simulink model "kinovaMicoSimscapeModel"  (R2021b)
settings: Solver=VariableStepAuto  StartTime=0.0  StopTime=0.3  FixedStep=0.01  RelTol=1e-3
PostLoadFcn:
  | micoRigidBodyTreeCreation;
  | IC=deg2rad([-90,180,180,0,0,0]);
  | interactiveHomePosition=deg2rad([-90 90 177.5 90 0 0]');
  | load("./KinovaMicoSimscapeVariantConfigurations.mat");
values from neighbouring files (symbols this model uses):
  micoCandlePosition = deg2rad([0,180,180,0,0,0])    [KinovaMicoSimscapeInitializeScript.m]    (also in generatingRandomTrajectory.m)
  ViaPointsTaskSpace = [ViaPointsTaskSpace;[[pi;0;pi],[pi;0;pi],[pi;0;pi],[pi;0;pi],[0;0;0],[0;0;0],[pi;0;pi]]]    [KinovaMicoSimscapeInitializeScript.m]    (also in generatingRandomTrajectory.m = [ViaPointsTaskSpace;zeros(3,7)])
undefined symbols (not defined in the file or in its folder): Mico, ViaPointsJointSpace, X, Y, Z
libraries: sm_lib x26, nesl_utility x19, robotcorelib x4, robotmaniplib x3, pid_lib x2
(part 2 of 50)

== system kinovaMicoSimscapeModel/StateErrorNorm/TaskSpaceError/Compute dqError ==
  dqd : Inport
  dq : Inport  Port=2
  Dot Product : DotProduct  InputSameDT=on  OutDataTypeStr=Inherit: Inherit via internal rule
  Sqrt : Sqrt  SaturateOnIntegerOverflow=on
  Subsystem : Subsystem  Commented=on
  Sum : Sum  Inputs=|+-
  dq_error : Outport
  wires:
  Sqrt/1 -> dq_error/1
  dq/1 -> Sum/2
  dqd/1 -> Sum/1
  Dot Product/1 -> Sqrt/1
  Sum/1 -> Dot Product/1, Dot Product/2

== system kinovaMicoSimscapeModel/StateErrorNorm/TaskSpaceError/Compute qError ==
  qd : Inport
  q : Inport  Port=2
  Dot Product : DotProduct  InputSameDT=on  OutDataTypeStr=Inherit: Inherit via internal rule
  Sqrt : Sqrt  SaturateOnIntegerOverflow=on
  Sum : Sum  Inputs=|+-
  q_error : Outport
  wires:
  Sum/1 -> Dot Product/2, Dot Product/1
  Dot Product/1 -> Sqrt/1
  qd/1 -> Sum/1
  q/1 -> Sum/2
  Sqrt/1 -> q_error/1

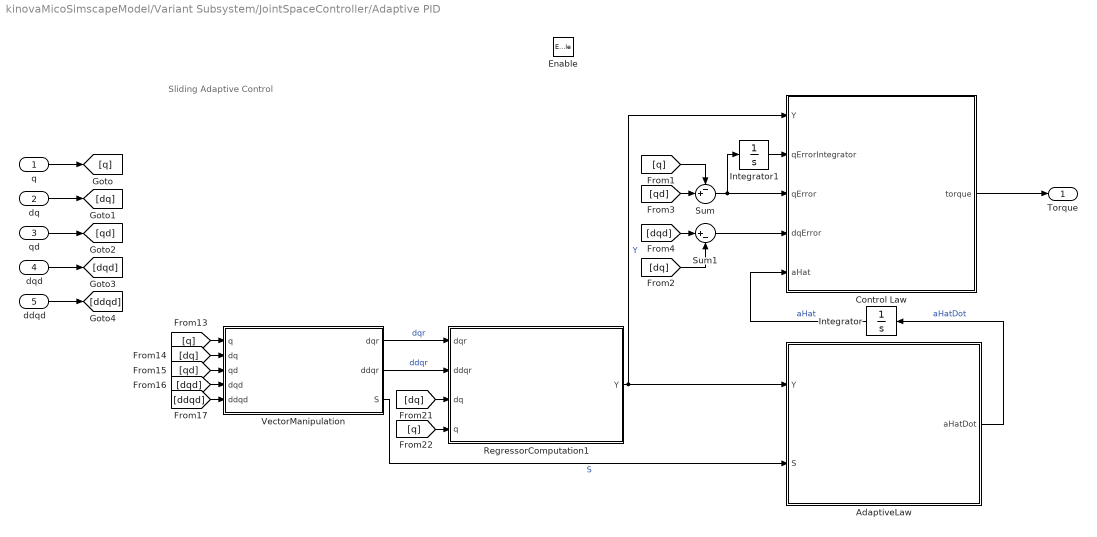
== system kinovaMicoSimscapeModel/Variant Subsystem/JointSpaceController/Adaptive PID ==
  note: Sliding Adaptive Control
  q : Inport
  dq : Inport  Port=2
  qd : Inport  Port=3
  dqd : Inport  Port=4
  ddqd : Inport  Port=5
  Enable : EnablePort
  AdaptiveLaw : MATLAB Function  TreatAsAtomicUnit=on
  Control Law : MATLAB Function  TreatAsAtomicUnit=on
  Integrator : Integrator
  Integrator1 : Integrator
  RegressorComputation1 : MATLAB Function  TreatAsAtomicUnit=on
  Sum : Sum  Inputs=-+|
  Sum1 : Sum  Inputs=|+-
  VectorManipulation : MATLAB Function  TreatAsAtomicUnit=on
  Torque : Outport
  wires:
  VectorManipulation/2(ddqr) -> RegressorComputation1/2(ddqr)  "ddqr"
  [qd] -> VectorManipulation/3(qd)
  VectorManipulation/3(S) -> AdaptiveLaw/2(S)  "S"
  [dqd] -> VectorManipulation/4(dqd)
  [ddqd] -> VectorManipulation/5(ddqd)
  [dq] -> RegressorComputation1/3(dq)
  [q] -> VectorManipulation/1(q)
  RegressorComputation1/1(Y) -> AdaptiveLaw/1(Y), Control Law/1(Y)  "Y"
  [dq] -> VectorManipulation/2(dq)
  Integrator/1 -> Control Law/5(aHat)  "aHat"
  [q] -> RegressorComputation1/4(q)
  VectorManipulation/1(dqr) -> RegressorComputation1/1(dqr)  "dqr"
  AdaptiveLaw/1(aHatDot) -> Integrator/1  "aHatDot"
  Control Law/1(torque) -> Torque/1
  q/1 -> [q]
  dq/1 -> [dq]
  qd/1 -> [qd]
  dqd/1 -> [dqd]
  ddqd/1 -> [ddqd]
  Sum/1 -> Integrator1/1, Control Law/3(qError)
  Integrator1/1 -> Control Law/2(qErrorIntegrator)
  [qd] -> Sum/2
  [q] -> Sum/1
  [dqd] -> Sum1/1
  [dq] -> Sum1/2
  Sum1/1 -> Control Law/4(dqError)

== system kinovaMicoSimscapeModel/Variant Subsystem/JointSpaceController/Enabled Subsystem ==
  q : Inport
  G_RNE : MATLAB Function  TreatAsAtomicUnit=on
  G : Outport
  wires:
  q/1 -> G_RNE/1(q)
  G_RNE/1(G) -> G/1  "gravity"

== system kinovaMicoSimscapeModel/Variant Subsystem/JointSpaceController/HybridImpedanceVelocityControl ==
  q : Inport
  dq : Inport  Port=2
  ddq : Inport  Port=3
  qd : Inport  Port=4
  dqd : Inport  Port=5
  ddqd : Inport  Port=6
  f : Inport  Port=7
  G : Inport  Port=8
  Enable : EnablePort
  C_RNE_SKEWSYMETRIC : MATLAB Function  TreatAsAtomicUnit=on
  Display : Display
  H_RNE : MATLAB Function  TreatAsAtomicUnit=on
  Hybrid Impedance Velocity Control : MATLAB Function  TreatAsAtomicUnit=on
  torque : Outport
  wires:
  ddq/1 -> Hybrid Impedance Velocity Control/3(ddq)
  Hybrid Impedance Velocity Control/1(torque) -> torque/1
  q/1 -> [q], Hybrid Impedance Velocity Control/1(q)
  dq/1 -> [dq], Hybrid Impedance Velocity Control/2(dq)
  qd/1 -> Hybrid Impedance Velocity Control/4(qd)
  dqd/1 -> Hybrid Impedance Velocity Control/5(dqd)
  ddqd/1 -> Hybrid Impedance Velocity Control/6(ddqd)
  f/1 -> Hybrid Impedance Velocity Control/7(f)
  H_RNE/1(M) -> Hybrid Impedance Velocity Control/8(H)  "mass"
  [q] -> H_RNE/1(q), C_RNE_SKEWSYMETRIC/1(q)
  [dq] -> C_RNE_SKEWSYMETRIC/2(dq)
  C_RNE_SKEWSYMETRIC/1(C) -> Hybrid Impedance Velocity Control/9(C)
  G/1 -> Hybrid Impedance Velocity Control/10(G)
  Hybrid Impedance Velocity Control/2(test) -> Display/1

== system kinovaMicoSimscapeModel/Variant Subsystem/JointSpaceController/Inverse Dynamics ==
  note: Inverse Dynamics
  q : Inport
  dq : Inport  Port=2
  qd : Inport  Port=3
  dqd : Inport  Port=4
  ddqd : Inport  Port=5
  G : Inport  Port=6
  Enable : EnablePort
  C_RNE_SKEWSYMETRIC : MATLAB Function  TreatAsAtomicUnit=on
  H_RNE : MATLAB Function  TreatAsAtomicUnit=on
  Inverse Dynamics : MATLAB Function  TreatAsAtomicUnit=on
  Matrix Multiply : Product  Multiplication=Matrix(*)
  Torque : Outport
  wires:
  ddqd/1 -> [ddqd]
  dqd/1 -> [dqd]
  qd/1 -> [qd]
  dq/1 -> [dq]
  q/1 -> [q]
  Inverse Dynamics/1(torque) -> Torque/1  "ComputedTorque"
  [q] -> H_RNE/1(q), C_RNE_SKEWSYMETRIC/1(q)
  [dq] -> C_RNE_SKEWSYMETRIC/2(dq)
  C_RNE_SKEWSYMETRIC/1(C) -> Matrix Multiply/1
  [dq] -> Matrix Multiply/2
  [q] -> Inverse Dynamics/4(q)
  [dq] -> Inverse Dynamics/5(dq)
  [qd] -> Inverse Dynamics/6(qd)
  [dqd] -> Inverse Dynamics/7(dqd)
  [ddqd] -> Inverse Dynamics/8(ddqd)
  H_RNE/1(M) -> Inverse Dynamics/1(M)  "mass"
  Matrix Multiply/1 -> Inverse Dynamics/2(Cdq)  "customCdq"
  G/1 -> Inverse Dynamics/3(G)

== system kinovaMicoSimscapeModel/Variant Subsystem/JointSpaceController/PD + Gravity ==
  note: Inputs
  note: PD + Gravity Controller
  q : Inport
  dq : Inport  Port=2
  qd : Inport  Port=3
  dqd : Inport  Port=4
  ddqd : Inport  Port=5
  G : Inport  Port=6
  Enable : EnablePort
  Gain : Gain  Gain=diag([25 25 25 15 15 15])  Multiplication=Matrix(K*u)
  Gain2 : Gain  Gain=diag([5 5 5 2 2 2])  Multiplication=Matrix(K*u)
  Sum : Sum  Inputs=|+-
  Sum1 : Sum  Inputs=|++
  Sum3 : Sum  Inputs=|+-
  Terminator : Terminator
  Terminator2 : Terminator
  Torque : Outport
  wires:
  Sum1/1 -> Torque/1
  dqd/1 -> Terminator2/1
  ddqd/1 -> Terminator/1
  qd/1 -> [qd]
  dq/1 -> [dq]
  q/1 -> [q]
  [q] -> Sum/2
  [dq] -> Gain2/1
  [qd] -> Sum/1
  Sum/1 -> Gain/1
  Gain/1 -> Sum3/1
  Gain2/1 -> Sum3/2
  Sum3/1 -> Sum1/1
  G/1 -> Sum1/2  "gravity"

== system kinovaMicoSimscapeModel/Variant Subsystem/JointSpaceController/PID ==
  note: Damping + Gravity Controller
  q : Inport
  dq : Inport  Port=2
  qd : Inport  Port=3
  dqd : Inport  Port=4
  ddqd : Inport  Port=5
  G : Inport  Port=6
  Enable : EnablePort
  Gain2 : Gain  Gain=0.1*ones(6,1)
  Gain3 : Gain  Gain=0.65*diag([25 25 25 8 8 8])  Multiplication=Matrix(K*u)
  Gain4 : Gain  Gain=0.25*diag([5 4 3 2 1.5 1.5])  Multiplication=Matrix(K*u)
  Integrator : Integrator
  Sum : Sum  Inputs=|+-
  Sum1 : Sum  Inputs=++++
  Sum2 : Sum  Inputs=|+-
  Terminator : Terminator
  Torque : Outport
  wires:
  Sum1/1 -> Torque/1
  dqd/1 -> [dqd]
  ddqd/1 -> Terminator/1
  qd/1 -> [qd]
  dq/1 -> [dq]
  q/1 -> [q]
  [qd] -> Sum/1
  [q] -> Sum/2
  [dqd] -> Sum2/1
  [dq] -> Sum2/2
  Sum/1 -> Gain3/1, Integrator/1
  Gain3/1 -> Sum1/2
  Sum2/1 -> Gain4/1
  Gain4/1 -> Sum1/3
  Integrator/1 -> Gain2/1
  Gain2/1 -> Sum1/1
  G/1 -> Sum1/4  "gravity"

== system kinovaMicoSimscapeModel/Variant Subsystem/JointSpaceController/Sliding Adaptive Control ==
  note: Sliding Adaptive Control
  q : Inport
  dq : Inport  Port=2
  qd : Inport  Port=3
  dqd : Inport  Port=4
  ddqd : Inport  Port=5
  Enable : EnablePort
  AdaptiveLaw : MATLAB Function  TreatAsAtomicUnit=on
  Control Law : MATLAB Function  TreatAsAtomicUnit=on
  Integrator : Integrator
  RegressorComputation : MATLAB Function  Commented=on  TreatAsAtomicUnit=on
  RegressorComputation1 : MATLAB Function  TreatAsAtomicUnit=on
  VectorManipulation : MATLAB Function  TreatAsAtomicUnit=on
  torqueDelayStuff : Subsystem  Commented=on
  Torque : Outport
  wires:
  ddqd/1 -> [ddqd]
  dqd/1 -> [dqd]
  qd/1 -> [qd]
  dq/1 -> [dq]
  q/1 -> [q]
  Control Law/1(torque) -> Torque/1  "AdaptiveTorque"
  AdaptiveLaw/1(aHatDot) -> Integrator/1  "aHatDot"
  VectorManipulation/2(dqr) -> RegressorComputation1/1(dqr)  "dqr"
  [q] -> RegressorComputation1/4(q)
  Integrator/1 -> Control Law/3(aHat)  "aHat"
  [dq] -> VectorManipulation/2(dq)
  RegressorComputation1/1(Y) -> Control Law/2(Y), AdaptiveLaw/1(Y)  "Y"
  [q] -> VectorManipulation/1(q)
  [dq] -> RegressorComputation1/3(dq)
  [ddqd] -> VectorManipulation/5(ddqd)
  [dqd] -> VectorManipulation/4(dqd)
  VectorManipulation/1(S) -> AdaptiveLaw/2(S), Control Law/1(S)  "S"
  [qd] -> VectorManipulation/3(qd)
  VectorManipulation/3(ddqr) -> RegressorComputation1/2(ddqr)  "ddqr"

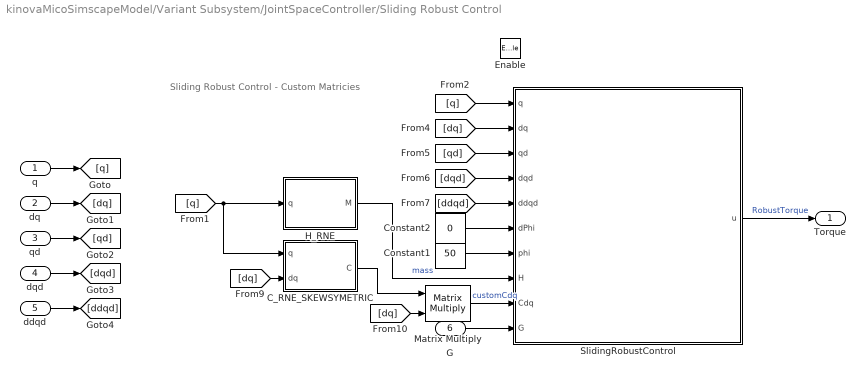
== system kinovaMicoSimscapeModel/Variant Subsystem/JointSpaceController/Sliding Robust Control ==
  note: Sliding Robust Control - Custom Matricies
  q : Inport
  dq : Inport  Port=2
  qd : Inport  Port=3
  dqd : Inport  Port=4
  ddqd : Inport  Port=5
  G : Inport  Port=6
  Enable : EnablePort
  C_RNE_SKEWSYMETRIC : MATLAB Function  TreatAsAtomicUnit=on
  Constant1 : Constant  Value=50
  Constant2 : Constant  Value=0
  H_RNE : MATLAB Function  TreatAsAtomicUnit=on
  Matrix Multiply : Product  Multiplication=Matrix(*)
  SlidingRobustControl : MATLAB Function  TreatAsAtomicUnit=on
  Torque : Outport
  wires:
  [dqd] -> SlidingRobustControl/4(dqd)
  [dq] -> Matrix Multiply/2
  C_RNE_SKEWSYMETRIC/1(C) -> Matrix Multiply/1
  Matrix Multiply/1 -> SlidingRobustControl/9(Cdq)  "customCdq"
  [qd] -> SlidingRobustControl/3(qd)
  [dq] -> C_RNE_SKEWSYMETRIC/2(dq)
  [ddqd] -> SlidingRobustControl/5(ddqd)
  Constant2/1 -> SlidingRobustControl/6(dPhi)
  [q] -> SlidingRobustControl/1(q)
  H_RNE/1(M) -> SlidingRobustControl/8(H)  "mass"
  Constant1/1 -> SlidingRobustControl/7(phi)
  [dq] -> SlidingRobustControl/2(dq)
  [q] -> H_RNE/1(q), C_RNE_SKEWSYMETRIC/1(q)
  SlidingRobustControl/1(u) -> Torque/1  "RobustTorque"
  q/1 -> [q]
  dq/1 -> [dq]
  qd/1 -> [qd]
  dqd/1 -> [dqd]
  ddqd/1 -> [ddqd]
  G/1 -> SlidingRobustControl/10(G)

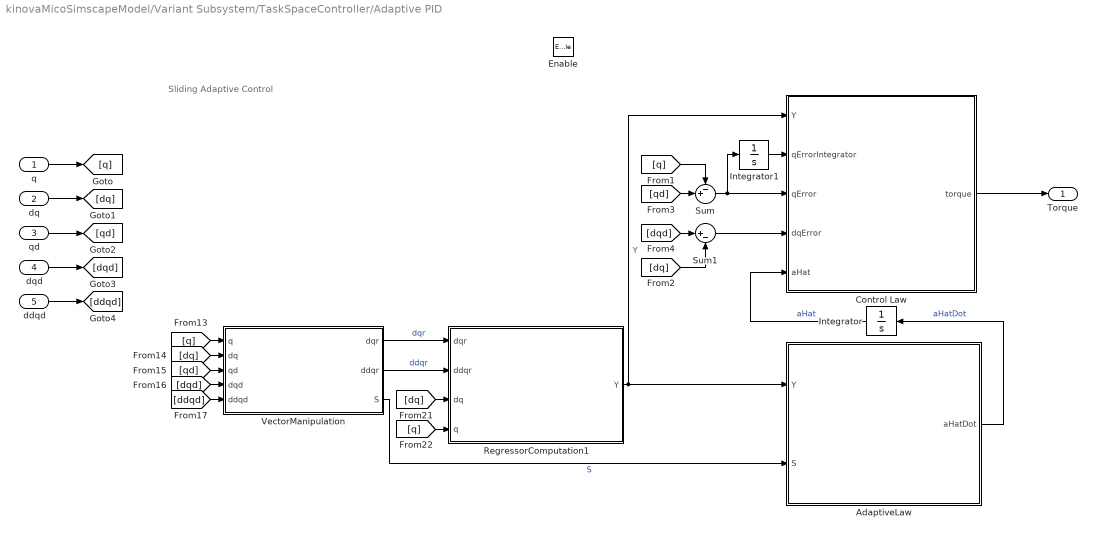
== system kinovaMicoSimscapeModel/Variant Subsystem/TaskSpaceController/Adaptive PID ==
  note: Sliding Adaptive Control
  q : Inport
  dq : Inport  Port=2
  qd : Inport  Port=3
  dqd : Inport  Port=4
  ddqd : Inport  Port=5
  Enable : EnablePort
  AdaptiveLaw : MATLAB Function  TreatAsAtomicUnit=on
  Control Law : MATLAB Function  TreatAsAtomicUnit=on
  Integrator : Integrator
  Integrator1 : Integrator
  RegressorComputation1 : MATLAB Function  TreatAsAtomicUnit=on
  Sum : Sum  Inputs=-+|
  Sum1 : Sum  Inputs=|+-
  VectorManipulation : MATLAB Function  TreatAsAtomicUnit=on
  Torque : Outport
  wires:
  Sum1/1 -> Control Law/4(dqError)
  [dq] -> Sum1/2
  [dqd] -> Sum1/1
  [q] -> Sum/1
  [qd] -> Sum/2
  Integrator1/1 -> Control Law/2(qErrorIntegrator)
  Sum/1 -> Control Law/3(qError), Integrator1/1
  ddqd/1 -> [ddqd]
  dqd/1 -> [dqd]
  qd/1 -> [qd]
  dq/1 -> [dq]
  q/1 -> [q]
  Control Law/1(torque) -> Torque/1
  AdaptiveLaw/1(aHatDot) -> Integrator/1  "aHatDot"
  VectorManipulation/1(dqr) -> RegressorComputation1/1(dqr)  "dqr"
  [q] -> RegressorComputation1/4(q)
  Integrator/1 -> Control Law/5(aHat)  "aHat"
  [dq] -> VectorManipulation/2(dq)
  RegressorComputation1/1(Y) -> Control Law/1(Y), AdaptiveLaw/1(Y)  "Y"
  [q] -> VectorManipulation/1(q)
  [dq] -> RegressorComputation1/3(dq)
  [ddqd] -> VectorManipulation/5(ddqd)
  [dqd] -> VectorManipulation/4(dqd)
  VectorManipulation/3(S) -> AdaptiveLaw/2(S)  "S"
  [qd] -> VectorManipulation/3(qd)
  VectorManipulation/2(ddqr) -> RegressorComputation1/2(ddqr)  "ddqr"

== system kinovaMicoSimscapeModel/Variant Subsystem/TaskSpaceController/Enabled Subsystem ==
  q : Inport
  G_RNE : MATLAB Function  TreatAsAtomicUnit=on
  G : Outport
  wires:
  G_RNE/1(G) -> G/1  "gravity"
  q/1 -> G_RNE/1(q)

== system kinovaMicoSimscapeModel/Variant Subsystem/TaskSpaceController/HybridImpedanceVelocityControl ==
  q : Inport
  dq : Inport  Port=2
  ddq : Inport  Port=3
  qd : Inport  Port=4
  dqd : Inport  Port=5
  ddqd : Inport  Port=6
  f : Inport  Port=7
  G : Inport  Port=8
  Enable : EnablePort
  C_RNE_SKEWSYMETRIC : MATLAB Function  TreatAsAtomicUnit=on
  Display : Display
  H_RNE : MATLAB Function  TreatAsAtomicUnit=on
  Hybrid Impedance Velocity Control : MATLAB Function  TreatAsAtomicUnit=on
  torque : Outport
  wires:
  Hybrid Impedance Velocity Control/2(test) -> Display/1
  G/1 -> Hybrid Impedance Velocity Control/10(G)
  C_RNE_SKEWSYMETRIC/1(C) -> Hybrid Impedance Velocity Control/9(C)
  [dq] -> C_RNE_SKEWSYMETRIC/2(dq)
  [q] -> C_RNE_SKEWSYMETRIC/1(q), H_RNE/1(q)
  H_RNE/1(M) -> Hybrid Impedance Velocity Control/8(H)  "mass"
  f/1 -> Hybrid Impedance Velocity Control/7(f)
  ddqd/1 -> Hybrid Impedance Velocity Control/6(ddqd)
  dqd/1 -> Hybrid Impedance Velocity Control/5(dqd)
  qd/1 -> Hybrid Impedance Velocity Control/4(qd)
  dq/1 -> Hybrid Impedance Velocity Control/2(dq), [dq]
  q/1 -> Hybrid Impedance Velocity Control/1(q), [q]
  Hybrid Impedance Velocity Control/1(torque) -> torque/1
  ddq/1 -> Hybrid Impedance Velocity Control/3(ddq)

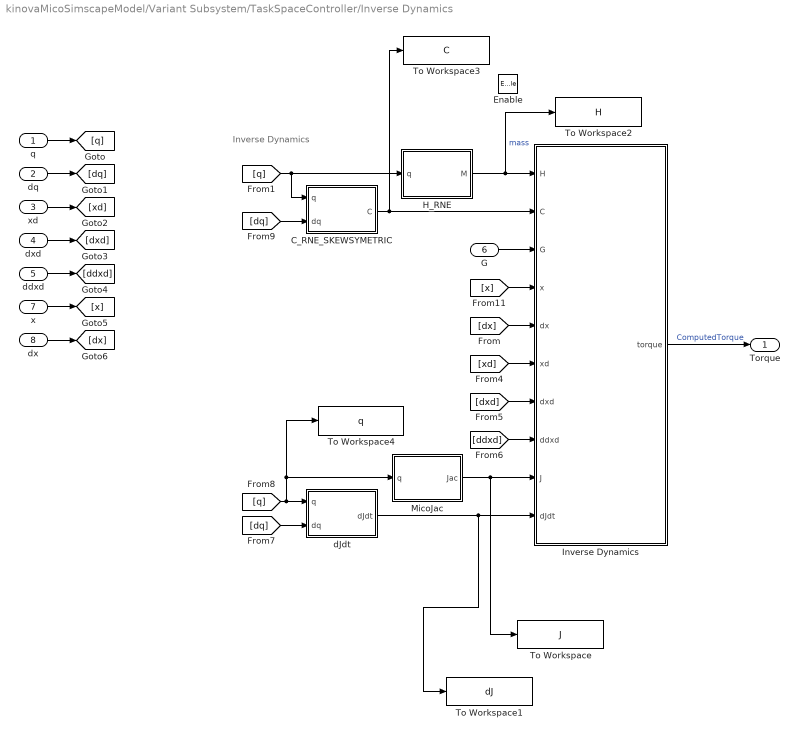
== system kinovaMicoSimscapeModel/Variant Subsystem/TaskSpaceController/Inverse Dynamics ==
  note: Inverse Dynamics
  q : Inport
  dq : Inport  Port=2
  xd : Inport  Port=3
  dxd : Inport  Port=4
  ddxd : Inport  Port=5
  G : Inport  Port=6
  x : Inport  Port=7
  dx : Inport  Port=8
  Enable : EnablePort
  C_RNE_SKEWSYMETRIC : MATLAB Function  TreatAsAtomicUnit=on
  H_RNE : MATLAB Function  TreatAsAtomicUnit=on
  Inverse Dynamics : MATLAB Function  TreatAsAtomicUnit=on
  MicoJac : MATLAB Function  TreatAsAtomicUnit=on
  To Workspace : ToWorkspace  VariableName=J  SampleTime=-1
      settings: MaxDataPoints=1
  To Workspace1 : ToWorkspace  VariableName=dJ  SampleTime=-1
      settings: MaxDataPoints=1
  To Workspace2 : ToWorkspace  VariableName=H  SampleTime=-1
      settings: MaxDataPoints=1
  To Workspace3 : ToWorkspace  VariableName=C  SampleTime=-1
      settings: MaxDataPoints=1
  To Workspace4 : ToWorkspace  VariableName=q  SampleTime=-1
      settings: MaxDataPoints=1
  dJdt : MATLAB Function  TreatAsAtomicUnit=on
  Torque : Outport
  wires:
  G/1 -> Inverse Dynamics/3(G)
  H_RNE/1(M) -> To Workspace2/1, Inverse Dynamics/1(H)  "mass"
  [ddxd] -> Inverse Dynamics/8(ddxd)
  [dxd] -> Inverse Dynamics/7(dxd)
  [xd] -> Inverse Dynamics/6(xd)
  [dq] -> C_RNE_SKEWSYMETRIC/2(dq)
  [q] -> C_RNE_SKEWSYMETRIC/1(q), H_RNE/1(q)
  q/1 -> [q]
  dq/1 -> [dq]
  xd/1 -> [xd]
  dxd/1 -> [dxd]
  ddxd/1 -> [ddxd]
  [dq] -> dJdt/2(dq)
  [q] -> To Workspace4/1, MicoJac/1(q), dJdt/1(q)
  x/1 -> [x]
  dx/1 -> [dx]
  [dx] -> Inverse Dynamics/5(dx)
  [x] -> Inverse Dynamics/4(x)
  MicoJac/1(Jac) -> To Workspace/1, Inverse Dynamics/9(J)
  dJdt/1(dJdt) -> To Workspace1/1, Inverse Dynamics/10(dJdt)
  C_RNE_SKEWSYMETRIC/1(C) -> Inverse Dynamics/2(C), To Workspace3/1
  Inverse Dynamics/1(torque) -> Torque/1  "ComputedTorque"

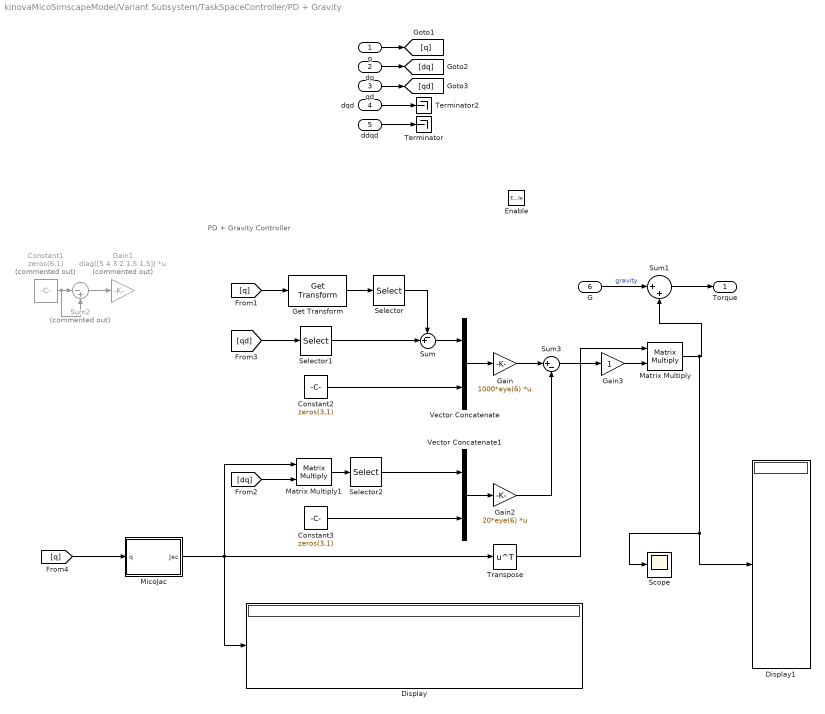
== system kinovaMicoSimscapeModel/Variant Subsystem/TaskSpaceController/PD + Gravity ==
  note: PD + Gravity Controller
  q : Inport
  dq : Inport  Port=2
  qd : Inport  Port=3
  dqd : Inport  Port=4
  ddqd : Inport  Port=5
  G : Inport  Port=6
  Enable : EnablePort
  Constant1 : Constant  Commented=on  Value=zeros(6,1)
  Constant2 : Constant  Value=zeros(3,1)
  Constant3 : Constant  Value=zeros(3,1)
  Display : Display
  Display1 : Display
  Gain : Gain  Gain=1000*eye(6)  Multiplication=Matrix(K*u)
  Gain1 : Gain  Commented=on  Gain=diag([5 4 3 2 1.5 1.5])  Multiplication=Matrix(K*u)
  Gain2 : Gain  Gain=20*eye(6)  Multiplication=Matrix(K*u)
  Gain3 : Gain
  Get Transform : robotmaniplib/Get Transform  RigidBodyTree=mico  SourceBody=EE  TargetBody=base  SimulateUsing=Code generation
  Matrix Multiply : Product  Multiplication=Matrix(*)
  Matrix Multiply1 : Product  Multiplication=Matrix(*)
  MicoJac : MATLAB Function  TreatAsAtomicUnit=on
  Scope : Scope
  Selector : Selector  NumberOfDimensions=2  InputPortWidth=3  IndexOptions=Index vector (dialog),Index vector (dialog)  Indices=[1:3],4  OutputSizes=1,1
  Selector1 : Selector  InputPortWidth=6  IndexOptions=Index vector (dialog)  Indices=[1:3]  OutputSizes=1
  Selector2 : Selector  InputPortWidth=6  IndexOptions=Index vector (dialog)  Indices=[1:3]  OutputSizes=1
  Sum : Sum  Inputs=-+|
  Sum1 : Sum  Inputs=|++
  Sum2 : Sum  Commented=on  Inputs=|-+
  Sum3 : Sum  Inputs=|+-
  Terminator : Terminator
  Terminator2 : Terminator
  Transpose : Math  Operator=transpose  SaturateOnIntegerOverflow=on
  Vector Concatenate : Concatenate
  Vector Concatenate1 : Concatenate
  Torque : Outport
  wires:
  Transpose/1 -> Matrix Multiply/1
  Gain3/1 -> Matrix Multiply/2
  Matrix Multiply/1 -> Sum1/2, Display1/1, Scope/1
  Gain/1 -> Sum3/1
  Gain2/1 -> Sum3/2
  Sum3/1 -> Gain3/1
  Selector2/1 -> Vector Concatenate1/1
  Matrix Multiply1/1 -> Selector2/1
  [dq] -> Matrix Multiply1/2
  Constant3/1 -> Vector Concatenate1/2
  Vector Concatenate1/1 -> Gain2/1
  Selector1/1 -> Sum/2
  [qd] -> Selector1/1
  G/1 -> Sum1/1  "gravity"
  MicoJac/1(Jac) -> Matrix Multiply1/1, Transpose/1, Display/1
  Vector Concatenate/1 -> Gain/1
  Constant2/1 -> Vector Concatenate/2
  Sum/1 -> Vector Concatenate/1
  [q] -> MicoJac/1(q)
  Selector/1 -> Sum/1
  Get Transform/1 -> Selector/1
  [q] -> Get Transform/1
  Constant1/1 -> Sum2/1, Sum2/2
  q/1 -> [q]
  dq/1 -> [dq]
  qd/1 -> [qd]
  ddqd/1 -> Terminator/1
  dqd/1 -> Terminator2/1
  Sum2/1 -> Gain1/1
  Sum1/1 -> Torque/1

== system kinovaMicoSimscapeModel/Variant Subsystem/TaskSpaceController/PID ==
  note: Damping + Gravity Controller
  q : Inport
  dq : Inport  Port=2
  qd : Inport  Port=3
  dqd : Inport  Port=4
  ddqd : Inport  Port=5
  G : Inport  Port=6
  Enable : EnablePort
  Gain2 : Gain  Gain=0.1*ones(6,1)
  Gain3 : Gain  Gain=0.65*diag([25 25 25 8 8 8])  Multiplication=Matrix(K*u)
  Gain4 : Gain  Gain=0.25*diag([5 4 3 2 1.5 1.5])  Multiplication=Matrix(K*u)
  Integrator : Integrator
  Sum : Sum  Inputs=|+-
  Sum1 : Sum  Inputs=++++
  Sum2 : Sum  Inputs=|+-
  Terminator : Terminator
  Terminator2 : Terminator
  Torque : Outport
  wires:
  G/1 -> Sum1/4  "gravity"
  Gain2/1 -> Sum1/1
  Integrator/1 -> Gain2/1
  Gain4/1 -> Sum1/3
  Sum2/1 -> Gain4/1
  Gain3/1 -> Sum1/2
  Sum/1 -> Integrator/1, Gain3/1
  [dq] -> Sum2/2
  [dqd] -> Sum2/1
  [q] -> Sum/2
  [qd] -> Sum/1
  q/1 -> [q]
  dq/1 -> [dq]
  qd/1 -> [qd]
  ddqd/1 -> Terminator/1
  dqd/1 -> Terminator2/1
  Sum1/1 -> Torque/1

== system kinovaMicoSimscapeModel/Variant Subsystem/TaskSpaceController/Sliding Adaptive Control ==
  note: Sliding Adaptive Control
  q : Inport
  dq : Inport  Port=2
  qd : Inport  Port=3
  dqd : Inport  Port=4
  ddqd : Inport  Port=5
  Enable : EnablePort
  AdaptiveLaw : MATLAB Function  TreatAsAtomicUnit=on
  Control Law : MATLAB Function  TreatAsAtomicUnit=on
  Integrator : Integrator
  RegressorComputation : MATLAB Function  Commented=on  TreatAsAtomicUnit=on
  RegressorComputation1 : MATLAB Function  TreatAsAtomicUnit=on
  VectorManipulation : MATLAB Function  TreatAsAtomicUnit=on
  torqueDelayStuff : Subsystem  Commented=on
  Torque : Outport
  wires:
  VectorManipulation/3(ddqr) -> RegressorComputation1/2(ddqr)  "ddqr"
  [qd] -> VectorManipulation/3(qd)
  VectorManipulation/1(S) -> Control Law/1(S), AdaptiveLaw/2(S)  "S"
  [dqd] -> VectorManipulation/4(dqd)
  [ddqd] -> VectorManipulation/5(ddqd)
  [dq] -> RegressorComputation1/3(dq)
  [q] -> VectorManipulation/1(q)
  RegressorComputation1/1(Y) -> Control Law/2(Y), AdaptiveLaw/1(Y)  "Y"
  [dq] -> VectorManipulation/2(dq)
  Integrator/1 -> Control Law/3(aHat)  "aHat"
  [q] -> RegressorComputation1/4(q)
  VectorManipulation/2(dqr) -> RegressorComputation1/1(dqr)  "dqr"
  AdaptiveLaw/1(aHatDot) -> Integrator/1  "aHatDot"
  Control Law/1(torque) -> Torque/1  "AdaptiveTorque"
  q/1 -> [q]
  dq/1 -> [dq]
  qd/1 -> [qd]
  dqd/1 -> [dqd]
  ddqd/1 -> [ddqd]

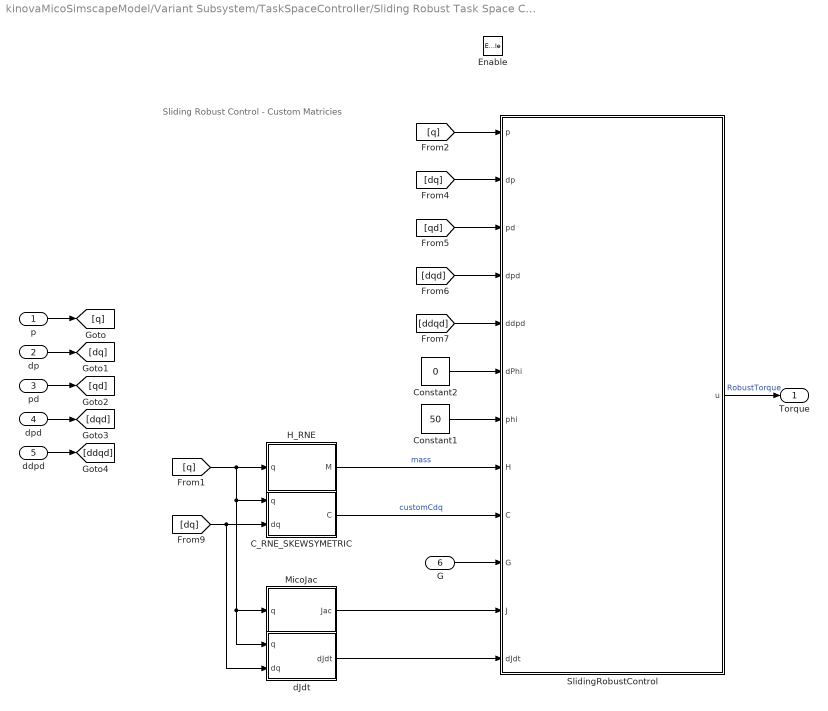
== system kinovaMicoSimscapeModel/Variant Subsystem/TaskSpaceController/Sliding Robust Task Space Control ==
  note: Sliding Robust Control - Custom Matricies
  p : Inport
  dp : Inport  Port=2
  pd : Inport  Port=3
  dpd : Inport  Port=4
  ddpd : Inport  Port=5
  G : Inport  Port=6
  Enable : EnablePort
  C_RNE_SKEWSYMETRIC : MATLAB Function  TreatAsAtomicUnit=on
  Constant1 : Constant  Value=50
  Constant2 : Constant  Value=0
  H_RNE : MATLAB Function  TreatAsAtomicUnit=on
  MicoJac : MATLAB Function  TreatAsAtomicUnit=on
  SlidingRobustControl : MATLAB Function  TreatAsAtomicUnit=on
  dJdt : MATLAB Function  TreatAsAtomicUnit=on
  Torque : Outport
  wires:
  MicoJac/1(Jac) -> SlidingRobustControl/11(J)
  dJdt/1(dJdt) -> SlidingRobustControl/12(dJdt)
  G/1 -> SlidingRobustControl/10(G)
  ddpd/1 -> [ddqd]
  dpd/1 -> [dqd]
  pd/1 -> [qd]
  dp/1 -> [dq]
  p/1 -> [q]
  SlidingRobustControl/1(u) -> Torque/1  "RobustTorque"
  [q] -> dJdt/1(q), MicoJac/1(q), C_RNE_SKEWSYMETRIC/1(q), H_RNE/1(q)
  [dq] -> SlidingRobustControl/2(dp)
  Constant1/1 -> SlidingRobustControl/7(phi)
  H_RNE/1(M) -> SlidingRobustControl/8(H)  "mass"
  [q] -> SlidingRobustControl/1(p)
  Constant2/1 -> SlidingRobustControl/6(dPhi)
  [ddqd] -> SlidingRobustControl/5(ddpd)
  [dq] -> C_RNE_SKEWSYMETRIC/2(dq), dJdt/2(dq)
  [qd] -> SlidingRobustControl/3(pd)
  C_RNE_SKEWSYMETRIC/1(C) -> SlidingRobustControl/9(C)  "customCdq"
  [dqd] -> SlidingRobustControl/4(dpd)

== system kinovaMicoSimscapeModel/StateErrorNorm/JointSpaceError/Compute dqError/Subsystem ==
  In1 : Inport
  Demux : Demux  Outputs=6
  Mux : Mux  Inputs=6
  Transfer Fcn{,1..5} (6 alike) : TransferFcn  Denominator=[1e-6 1]
  Out1 : Outport
  wires:
  Transfer Fcn1/1 -> Mux/2
  Demux/4 -> Transfer Fcn3/1
  Transfer Fcn2/1 -> Mux/3
  Demux/1 -> Transfer Fcn/1
  Transfer Fcn/1 -> Mux/1
  Demux/2 -> Transfer Fcn1/1
  Transfer Fcn4/1 -> Mux/5
  Mux/1 -> Out1/1
  In1/1 -> Demux/1
  Transfer Fcn5/1 -> Mux/6
  Demux/5 -> Transfer Fcn4/1
  Demux/3 -> Transfer Fcn2/1
  Demux/6 -> Transfer Fcn5/1
  Transfer Fcn3/1 -> Mux/4

== system kinovaMicoSimscapeModel/StateErrorNorm/JointSpaceError/Compute qError/Subsystem ==
  In1 : Inport
  Demux : Demux  Outputs=6
  Mux : Mux  Inputs=6
  Transfer Fcn{,1..5} (6 alike) : TransferFcn  Denominator=[1e-6 1]
  Out1 : Outport
  wires:
  Transfer Fcn3/1 -> Mux/4
  Demux/6 -> Transfer Fcn5/1
  Demux/3 -> Transfer Fcn2/1
  Demux/5 -> Transfer Fcn4/1
  Transfer Fcn5/1 -> Mux/6
  In1/1 -> Demux/1
  Mux/1 -> Out1/1
  Transfer Fcn4/1 -> Mux/5
  Demux/2 -> Transfer Fcn1/1
  Transfer Fcn/1 -> Mux/1
  Demux/1 -> Transfer Fcn/1
  Transfer Fcn2/1 -> Mux/3
  Demux/4 -> Transfer Fcn3/1
  Transfer Fcn1/1 -> Mux/2

== system kinovaMicoSimscapeModel/StateErrorNorm/TaskSpaceError/Compute dqError/Subsystem ==
  In1 : Inport
  Demux : Demux  Outputs=6
  Mux : Mux  Inputs=6
  Transfer Fcn{,1..5} (6 alike) : TransferFcn  Denominator=[1e-6 1]
  Out1 : Outport
  wires:
  Transfer Fcn1/1 -> Mux/2
  Demux/4 -> Transfer Fcn3/1
  Transfer Fcn2/1 -> Mux/3
  Demux/1 -> Transfer Fcn/1
  Transfer Fcn/1 -> Mux/1
  Demux/2 -> Transfer Fcn1/1
  Transfer Fcn4/1 -> Mux/5
  Mux/1 -> Out1/1
  In1/1 -> Demux/1
  Transfer Fcn5/1 -> Mux/6
  Demux/5 -> Transfer Fcn4/1
  Demux/3 -> Transfer Fcn2/1
  Demux/6 -> Transfer Fcn5/1
  Transfer Fcn3/1 -> Mux/4

== system kinovaMicoSimscapeModel/Variant Subsystem/JointSpaceController/Sliding Adaptive Control/torqueDelayStuff ==
  torque : Inport
  PID Controller1 : pid_lib/PID Controller  Controller=PID  Form=Parallel  TimeDomain=Continuous-time  UseExternalTs=off  SampleTime=-1  IntegratorMethod=Forward Euler  FilterMethod=Forward Euler  ControllerParametersSource=internal  P=5  I=0  D=1  UseFilter=on  N=100  TunerSelectOption=Transfer Function Based (PID Tuner App)  InitialConditionSource=internal  InitialConditionForIntegrator=0  InitialConditionForFilter=0  DifferentiatorICPrevScaledInput=0  ExternalReset=none  TrackingMode=off  Kt=1  LimitOutput=on  SatLimitsSource=internal  UpperSaturationLimit=2  LowerSaturationLimit=-2  LinearizeAsGain=on  AntiWindupMode=none  Kb=1  POutMin=[]  POutMax=[]  IOutMin=[]  IOutMax=[]  DOutMin=[]  DOutMax=[]  NOutMin=[]  NOutMax=[]  SumOutMin=[]  SumOutMax=[]  SaturationOutMin=[]  SaturationOutMax=[]  PParamMin=[]  PParamMax=[]  IParamMin=[]  IParamMax=[]  DParamMin=[]  DParamMax=[]  NParamMin=[]  NParamMax=[]  KbParamMin=[]  KbParamMax=[]  KtParamMin=[]  KtParamMax=[]  KbOutMin=[]  KbOutMax=[]  KtOutMin=[]  KtOutMax=[]  IntegratorOutMin=[]  IntegratorOutMax=[]  FilterOutMin=[]  FilterOutMax=[]  SumI1OutMin=[]  SumI1OutMax=[]  SumI2OutMin=[]  SumI2OutMax=[]  SumI3OutMin=[]  SumI3OutMax=[]  SumI4OutMin=[]  SumI4OutMax=[]  SumDOutMin=[]  SumDOutMax=[]  DifferentiatorOutMin=[]  DifferentiatorOutMax=[]  FilterDiffOutCoefMin=[]  FilterDiffOutCoefMax=[]  ReciprocalOutMin=[]  ReciprocalOutMax=[]  SumDenOutMin=[]  SumDenOutMax=[]  SumNumOutMin=[]  SumNumOutMax=[]  DivideOutMin=[]  DivideOutMax=[]  UdiffTsProdOutMin=[]  UdiffTsProdOutMax=[]  NTsProdOutMin=[]  NTsProdOutMax=[]  UintegralTsProdOutMin=[]  UintegralTsProdOutMax=[]  UngainTsProdOutMin=[]  UngainTsProdOutMax=[]  IntegratorContinuousStateAttributes=''  IntegratorStateMustResolveToSignalObject=off  IntegratorRTWStateStorageClass=Auto  FilterContinuousStateAttributes=''  FilterStateMustResolveToSignalObject=off  FilterRTWStateStorageClass=Auto  ParallelPVariant=InternalParameters  IdealPVariant=Disabled  IVariant=InternalParameters  DVariant=InternalParameters  IntegratorVariant=Continuous  SatVariant=Enabled  AWVariant=Passthrough  PCopyVariant=Disabled  TRVariant=Disabled  FdbkBlocksVariant=Forward  IdealPFdbkVariant=Disabled  SatFdbkVariant=Disabled  DerivativeFilterVariant=ContFilter  NVariant=InternalParameters  NCopyVariant=Disabled  FilterICVariant=InternalICsFilter  IntegratorICVariant=InternalICs  ExternalResetVariant=Disabled  TRSumVariant=Passthrough  SumFdbkVariant=Disabled  SumVariant=Sum_PID  TsampFilterVariant=InternalTs  TsampNgainVariant=Passthrough  TsampIntegralVariant=Passthrough  ExternalSaturationOutDataTypeStr=Inherit: Same as second input
  Rate Transition : RateTransition  OutPortSampleTime=.01
  Rate Transition1 : RateTransition  OutPortSampleTime=.01
  Sum : Sum  Inputs=|+-
  transferFunctionModelingPlant : Subsystem
  transferFunctionModelingPlant1 : Subsystem
  Outport : Outport
  wires:
  Sum/1 -> PID Controller1/1
  transferFunctionModelingPlant/1(Outport) -> Sum/2  "PID_Torques"
  PID Controller1/1 -> transferFunctionModelingPlant/1(In1)  "allJointsPID"
  Rate Transition/1 -> Sum/1
  torque/1 -> Rate Transition1/1
  Rate Transition1/1 -> transferFunctionModelingPlant1/1(In1)
  transferFunctionModelingPlant1/1(Outport) -> Outport/1  "PID_Torques"

== system kinovaMicoSimscapeModel/Variant Subsystem/TaskSpaceController/Sliding Adaptive Control/torqueDelayStuff ==
  torque : Inport
  PID Controller1 : pid_lib/PID Controller  Controller=PID  Form=Parallel  TimeDomain=Continuous-time  UseExternalTs=off  SampleTime=-1  IntegratorMethod=Forward Euler  FilterMethod=Forward Euler  ControllerParametersSource=internal  P=5  I=0  D=1  UseFilter=on  N=100  TunerSelectOption=Transfer Function Based (PID Tuner App)  InitialConditionSource=internal  InitialConditionForIntegrator=0  InitialConditionForFilter=0  DifferentiatorICPrevScaledInput=0  ExternalReset=none  TrackingMode=off  Kt=1  LimitOutput=on  SatLimitsSource=internal  UpperSaturationLimit=2  LowerSaturationLimit=-2  LinearizeAsGain=on  AntiWindupMode=none  Kb=1  POutMin=[]  POutMax=[]  IOutMin=[]  IOutMax=[]  DOutMin=[]  DOutMax=[]  NOutMin=[]  NOutMax=[]  SumOutMin=[]  SumOutMax=[]  SaturationOutMin=[]  SaturationOutMax=[]  PParamMin=[]  PParamMax=[]  IParamMin=[]  IParamMax=[]  DParamMin=[]  DParamMax=[]  NParamMin=[]  NParamMax=[]  KbParamMin=[]  KbParamMax=[]  KtParamMin=[]  KtParamMax=[]  KbOutMin=[]  KbOutMax=[]  KtOutMin=[]  KtOutMax=[]  IntegratorOutMin=[]  IntegratorOutMax=[]  FilterOutMin=[]  FilterOutMax=[]  SumI1OutMin=[]  SumI1OutMax=[]  SumI2OutMin=[]  SumI2OutMax=[]  SumI3OutMin=[]  SumI3OutMax=[]  SumI4OutMin=[]  SumI4OutMax=[]  SumDOutMin=[]  SumDOutMax=[]  DifferentiatorOutMin=[]  DifferentiatorOutMax=[]  FilterDiffOutCoefMin=[]  FilterDiffOutCoefMax=[]  ReciprocalOutMin=[]  ReciprocalOutMax=[]  SumDenOutMin=[]  SumDenOutMax=[]  SumNumOutMin=[]  SumNumOutMax=[]  DivideOutMin=[]  DivideOutMax=[]  UdiffTsProdOutMin=[]  UdiffTsProdOutMax=[]  NTsProdOutMin=[]  NTsProdOutMax=[]  UintegralTsProdOutMin=[]  UintegralTsProdOutMax=[]  UngainTsProdOutMin=[]  UngainTsProdOutMax=[]  IntegratorContinuousStateAttributes=''  IntegratorStateMustResolveToSignalObject=off  IntegratorRTWStateStorageClass=Auto  FilterContinuousStateAttributes=''  FilterStateMustResolveToSignalObject=off  FilterRTWStateStorageClass=Auto  ParallelPVariant=InternalParameters  IdealPVariant=Disabled  IVariant=InternalParameters  DVariant=InternalParameters  IntegratorVariant=Continuous  SatVariant=Enabled  AWVariant=Passthrough  PCopyVariant=Disabled  TRVariant=Disabled  FdbkBlocksVariant=Forward  IdealPFdbkVariant=Disabled  SatFdbkVariant=Disabled  DerivativeFilterVariant=ContFilter  NVariant=InternalParameters  NCopyVariant=Disabled  FilterICVariant=InternalICsFilter  IntegratorICVariant=InternalICs  ExternalResetVariant=Disabled  TRSumVariant=Passthrough  SumFdbkVariant=Disabled  SumVariant=Sum_PID  TsampFilterVariant=InternalTs  TsampNgainVariant=Passthrough  TsampIntegralVariant=Passthrough  ExternalSaturationOutDataTypeStr=Inherit: Same as second input
  Rate Transition : RateTransition  OutPortSampleTime=.01
  Rate Transition1 : RateTransition  OutPortSampleTime=.01
  Sum : Sum  Inputs=|+-
  transferFunctionModelingPlant : Subsystem
  transferFunctionModelingPlant1 : Subsystem
  Outport : Outport
  wires:
  transferFunctionModelingPlant1/1(Outport) -> Outport/1  "PID_Torques"
  Rate Transition1/1 -> transferFunctionModelingPlant1/1(In1)
  torque/1 -> Rate Transition1/1
  Rate Transition/1 -> Sum/1
  PID Controller1/1 -> transferFunctionModelingPlant/1(In1)  "allJointsPID"
  transferFunctionModelingPlant/1(Outport) -> Sum/2  "PID_Torques"
  Sum/1 -> PID Controller1/1

== system kinovaMicoSimscapeModel/Variant Subsystem/JointSpaceController/Sliding Adaptive Control/torqueDelayStuff/transferFunctionModelingPlant ==
  In1 : Inport
  Demux : Demux  Outputs=6
  Mux : Mux  Inputs=6
  Transfer Fcn{,1..5} (6 alike) : TransferFcn  Denominator=[1e-3 1]
  Outport : Outport
  wires:
  Demux/6 -> Transfer Fcn5/1
  Mux/1 -> Outport/1
  Transfer Fcn/1 -> Mux/1
  Transfer Fcn4/1 -> Mux/5
  Demux/2 -> Transfer Fcn1/1
  Transfer Fcn2/1 -> Mux/3
  Transfer Fcn1/1 -> Mux/2
  In1/1 -> Demux/1
  Transfer Fcn3/1 -> Mux/4
  Transfer Fcn5/1 -> Mux/6
  Demux/3 -> Transfer Fcn2/1
  Demux/4 -> Transfer Fcn3/1
  Demux/1 -> Transfer Fcn/1
  Demux/5 -> Transfer Fcn4/1

== system kinovaMicoSimscapeModel/Variant Subsystem/JointSpaceController/Sliding Adaptive Control/torqueDelayStuff/transferFunctionModelingPlant1 ==
  In1 : Inport
  Demux : Demux  Outputs=6
  Mux : Mux  Inputs=6
  Transfer Fcn{,1..5} (6 alike) : TransferFcn  Denominator=[1e-3 1]
  Outport : Outport
  wires:
  Demux/5 -> Transfer Fcn4/1
  Demux/1 -> Transfer Fcn/1
  Demux/4 -> Transfer Fcn3/1
  Demux/3 -> Transfer Fcn2/1
  Transfer Fcn5/1 -> Mux/6
  Transfer Fcn3/1 -> Mux/4
  In1/1 -> Demux/1
  Transfer Fcn1/1 -> Mux/2
  Transfer Fcn2/1 -> Mux/3
  Demux/2 -> Transfer Fcn1/1
  Transfer Fcn4/1 -> Mux/5
  Transfer Fcn/1 -> Mux/1
  Mux/1 -> Outport/1
  Demux/6 -> Transfer Fcn5/1

== system kinovaMicoSimscapeModel/Variant Subsystem/TaskSpaceController/Sliding Adaptive Control/torqueDelayStuff/transferFunctionModelingPlant ==
  In1 : Inport
  Demux : Demux  Outputs=6
  Mux : Mux  Inputs=6
  Transfer Fcn{,1..5} (6 alike) : TransferFcn  Denominator=[1e-3 1]
  Outport : Outport
  wires:
  Demux/5 -> Transfer Fcn4/1
  Demux/1 -> Transfer Fcn/1
  Demux/4 -> Transfer Fcn3/1
  Demux/3 -> Transfer Fcn2/1
  Transfer Fcn5/1 -> Mux/6
  Transfer Fcn3/1 -> Mux/4
  In1/1 -> Demux/1
  Transfer Fcn1/1 -> Mux/2
  Transfer Fcn2/1 -> Mux/3
  Demux/2 -> Transfer Fcn1/1
  Transfer Fcn4/1 -> Mux/5
  Transfer Fcn/1 -> Mux/1
  Mux/1 -> Outport/1
  Demux/6 -> Transfer Fcn5/1

== system kinovaMicoSimscapeModel/Variant Subsystem/TaskSpaceController/Sliding Adaptive Control/torqueDelayStuff/transferFunctionModelingPlant1 ==
  In1 : Inport
  Demux : Demux  Outputs=6
  Mux : Mux  Inputs=6
  Transfer Fcn{,1..5} (6 alike) : TransferFcn  Denominator=[1e-3 1]
  Outport : Outport
  wires:
  Demux/6 -> Transfer Fcn5/1
  Mux/1 -> Outport/1
  Transfer Fcn/1 -> Mux/1
  Transfer Fcn4/1 -> Mux/5
  Demux/2 -> Transfer Fcn1/1
  Transfer Fcn2/1 -> Mux/3
  Transfer Fcn1/1 -> Mux/2
  In1/1 -> Demux/1
  Transfer Fcn3/1 -> Mux/4
  Transfer Fcn5/1 -> Mux/6
  Demux/3 -> Transfer Fcn2/1
  Demux/4 -> Transfer Fcn3/1
  Demux/1 -> Transfer Fcn/1
  Demux/5 -> Transfer Fcn4/1

== matlab function kinovaMicoSimscapeModel/Variant Subsystem/JointSpaceController/Adaptive PID/AdaptiveLaw ==
  data: Y input; S input; aHatDot output
function aHatDot  = AdaptiveLaw(Y,S)
P=1500;
aHatDot=-P*transpose(Y)*S;

== matlab function kinovaMicoSimscapeModel/Variant Subsystem/JointSpaceController/Adaptive PID/Control Law ==
  data: Y input; qErrorIntegrator input; qError input; dqError input; aHat input; torque output
function torque  = AdaptiveControlLaw(Y,qErrorIntegrator,qError,dqError,aHat)
Kp=0*diag([2 2 2 1 1 1]);
Kv=0*diag([2 2 2 1 1 1]);
Ki=0*diag([1 1 1 1 1 1]);
torque=Y*aHat+Kp*qError+Kv*dqError+Ki*qErrorIntegrator;
